simulink model "Sim_Prob3_d"  (R2017b)
settings: Solver=FixedStepAuto  StartTime=0.0  StopTime=20.0  FixedStep=0.001  RelTol=1e-3
settings Model: Creator=Daslab  LastModifiedBy=thapa

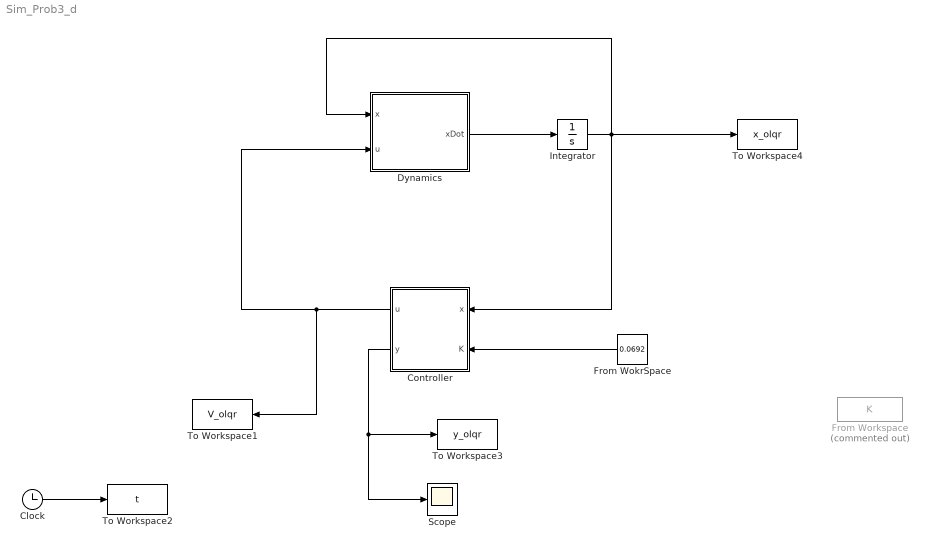
== system Sim_Prob3_d ==
  Clock : Clock
  Controller : MATLAB Function  TreatAsAtomicUnit=on
  Dynamics : MATLAB Function  TreatAsAtomicUnit=on
  From Workspace : FromWorkspace  Commented=on  VariableName=K  SampleTime=0
  From WokrSpace : Constant  Value=0.0692
  Integrator : Integrator  InitialCondition=[1;0.1;0]
  Scope : Scope
  To Workspace1 : ToWorkspace  VariableName=V_olqr  SampleTime=-1
      settings: Save2DSignal=2-D array (concatenate along first dimension)
  To Workspace2 : ToWorkspace  VariableName=t  SampleTime=-1
      settings: Save2DSignal=2-D array (concatenate along first dimension)
  To Workspace3 : ToWorkspace  VariableName=y_olqr  SampleTime=-1
      settings: Save2DSignal=2-D array (concatenate along first dimension)
  To Workspace4 : ToWorkspace  VariableName=x_olqr  SampleTime=-1
      settings: Save2DSignal=2-D array (concatenate along first dimension)
  wires:
  Dynamics/1(xDot) -> Integrator/1
  Integrator/1 -> Controller/1(x), Dynamics/1(x), To Workspace4/1
  Controller/1(u) -> To Workspace1/1, Dynamics/2(u)
  Clock/1 -> To Workspace2/1
  Controller/2(y) -> To Workspace3/1, Scope/1
  From WokrSpace/1 -> Controller/2(K)

== matlab function Sim_Prob3_d/Controller ==
  data: x input; u output; y output; K input
function [u,y] = Controller(x,K)
C = [0 1 1];
y = C*x;
u = -K*y;

== matlab function Sim_Prob3_d/Dynamics ==
  data: x input; u input; xDot output
function xDot = Dynamics(x,u)

Lp = -1; % rad/s
Ldela = 30; % s^-2; 
tau = 0.1; % sec 
% 
% Deldela_max = 0.436; % rad 
% Delphi_max = 0.787; % rad 
% delv_max = 10; % volts

A = [Lp 0 Ldela; 
     1  0 0; 
     0  0 -1/tau];

B = [0 0 1/tau]';

xDot = A*x + B*u;
